simulink model "AB_Final_of_MPC_Bandwidth_Result_UnbalancedNew"  (R2022b)
settings: Solver=FixedStepDiscrete  StartTime=0.0  StopTime=Inf  FixedStep=100e-6  RelTol=1e-3  EnableMultiTasking=on
undefined symbols (not defined in the file): C28x, CPU1, CPU2, CurrentBypassValue, DiscIntNeverNeededParam, Down, GPTRIP1SEL, TZ1, Up
libraries: c2802xlib x20, simulink x17, dspstat3 x13, eeGeneralControl x10, c2837xDlib x5, c280xlib x5, PID_Lib x4, c2000lib x1, spsAlphaBetaZerotoabcLib x1
(part 7 of 10)

== system AB_Final_of_MPC_Bandwidth_Result_UnbalancedNew/Subsystem1/dq_abc1/Subsystem6 ==
  In1 : Inport
  In2 : Inport  Port=2
  theta : Inport  Port=3
  Add{,1,3..4} (4 alike) : Sum  Inputs=+-
  Add2 : Sum
  Constant : Constant  Value=2*pi/3
  Cos : Trigonometry  Operator=cos
  Cos1 : Trigonometry
  Cos2 : Trigonometry  Operator=cos
  Cos3 : Trigonometry
  Cos4 : Trigonometry
  Cos5 : Trigonometry  Operator=cos
  Product{,1..5} (6 alike) : Product
  Ia : Outport
  Ib : Outport  Port=2
  Ic : Outport  Port=3
  wires:
  theta/1 -> Add2/2, Add3/1, Cos1/1, Cos/1
  In1/1 -> [d]
  In2/1 -> [q]
  [d] -> Product/1
  Cos/1 -> [cosine]
  Cos1/1 -> [sinee]
  [cosine] -> Product/2
  [q] -> Product1/1
  [sinee] -> Product1/2
  Product/1 -> Add/1
  Product1/1 -> Add/2
  Add/1 -> Ia/1
  Constant/1 -> Add3/2, Add2/1
  Add2/1 -> Cos4/1, Cos2/1
  Add3/1 -> Cos5/1, Cos3/1
  Add1/1 -> Ib/1
  [d] -> Product2/1
  Cos3/1 -> Product3/2
  Product3/1 -> Add1/2
  [q] -> Product3/1
  Product2/1 -> Add1/1
  Cos5/1 -> Product2/2
  [q] -> Product5/1
  [d] -> Product4/1
  Product4/1 -> Add4/1
  Add4/1 -> Ic/1
  Cos4/1 -> Product5/2
  Product5/1 -> Add4/2
  Cos2/1 -> Product4/2

== system AB_Final_of_MPC_Bandwidth_Result_UnbalancedNew/Subsystem3/PLL_Loop2/ABCtoAlphaBeta ==
  In1 : Inport
  In2 : Inport  Port=2
  In3 : Inport  Port=3
  Add : Sum  Inputs=+-
  Add1 : Sum  Inputs=+--
  Gain : Gain  Gain=0.5
  Gain1 : Gain  Gain=sqrt(3)/2
  Gain2 : Gain  Gain=2/3
  Gain3 : Gain  Gain=2/3
  Gain4 : Gain  Gain=0.5
  Out1 : Outport
  Vαβ : Outport  Port=2
  wires:
  In1/1 -> Add1/1
  Gain4/1 -> Add1/3
  Gain/1 -> Add1/2
  In2/1 -> Add/1, Gain/1
  In3/1 -> Add/2, Gain4/1
  Add/1 -> Gain1/1
  Add1/1 -> Gain2/1
  Gain2/1 -> Out1/1
  Gain1/1 -> Gain3/1
  Gain3/1 -> Vαβ/1

== system AB_Final_of_MPC_Bandwidth_Result_UnbalancedNew/Subsystem3/PLL_Loop2/Discrete integrator 2π wrapping1 ==
  ω : Inport
  Compare To Constant : simulink/Logic and Bit Operations/Compare To Constant  relop=<  const=0  OutDataTypeStr=boolean
  Compare To Constant1 : simulink/Logic and Bit Operations/Compare To Constant  relop=>=  const=2*pi  OutDataTypeStr=boolean
  Discrete-Time Integrator : DiscreteIntegrator  ExternalReset=sampled level  InitialConditionSource=external  SampleTime=-1  ShowStatePort=on  ICPrevOutput=DiscIntNeverNeededParam  ICPrevScaledInput=DiscIntNeverNeededParam
  Gain : Gain  Gain=1/(2*pi)
      settings: AttributesFormatString=%<Gain>
  Gain1 : Gain  Gain=2*pi
  IC : InitialCondition  Value=0
  Logical Operator : Logic  Operator=OR  AllPortsSameDT=off  OutDataTypeStr=boolean
  Rounding Function : Rounding
  Sum1 : Sum  Inputs=|+-
  θ : Outport
  wires:
  Gain1/1 -> Sum1/2
  Gain/1 -> Rounding Function/1
  IC/1 -> Discrete-Time Integrator/3
  Compare To Constant1/1 -> Logical Operator/2
  Discrete-Time Integrator/State -> Compare To Constant1/1, Sum1/1, Gain/1, Compare To Constant/1
  Compare To Constant/1 -> Logical Operator/1
  Logical Operator/1 -> Discrete-Time Integrator/2
  Sum1/1 -> IC/1
  Rounding Function/1 -> Gain1/1
  ω/1 -> Discrete-Time Integrator/1
  Discrete-Time Integrator/1 -> θ/1

== system AB_Final_of_MPC_Bandwidth_Result_UnbalancedNew/Subsystem3/PLL_Loop2/SOGI 1st2 ==
  w : Inport
  Vαβ : Inport  Port=2
  Cast To Single : DataTypeConversion  OutDataTypeStr=single  SaturateOnIntegerOverflow=off  RndMeth=Floor
  Delay One Step : Delay  DelayLength=1  InitialCondition=0.5
  Delay One Step1 : Delay  DelayLength=1  InitialCondition=-0.5
  Gain : Gain  Gain=sqrt(2)  OutDataTypeStr=single
  Gain1 : Gain  Gain=100e-6  OutDataTypeStr=single
  Multiply1 : Product
  Product : Product
  Sum : Sum  Inputs=-+|
  Sum1 : Sum  Inputs=|+-
  Sum2 : Sum  Inputs=++|
  Sum3 : Sum  Inputs=++|
  v : Outport
  qv : Outport  Port=2  OutDataTypeStr=single
  wires:
  Sum/1 -> Gain/1
  Gain/1 -> Sum1/1
  Vαβ/1 -> Sum/2
  w/1 -> Gain1/1
  Sum1/1 -> Product/2
  Gain1/1 -> [WTs], Product/1
  Product/1 -> Sum2/2
  Sum2/1 -> Cast To Single/1, Delay One Step/1, v/1
  Delay One Step/1 -> Sum2/1, Sum/1
  [WTs] -> Multiply1/2
  Multiply1/1 -> Sum3/2
  Delay One Step1/1 -> Sum3/1, Sum1/2
  Sum3/1 -> Delay One Step1/1, qv/1
  Cast To Single/1 -> Multiply1/1

== system AB_Final_of_MPC_Bandwidth_Result_UnbalancedNew/Subsystem3/PLL_Loop2/SOGI 1st3 ==
  w : Inport
  Vαβ : Inport  Port=2
  Gain : Gain  Gain=sqrt(2)  OutDataTypeStr=single
  Gain1 : Gain  Gain=0  OutDataTypeStr=single
  Integrator : Subsystem
  Integrator1 : Subsystem
  Integrator2 : Subsystem
  Multiply : Product
  Multiply1 : Product
  Multiply2 : Product
  Saturation : Saturate  UpperLimit=5  LowerLimit=-5
  Sum : Sum  Inputs=-+|
  Sum1 : Sum  Inputs=|+-
  Sum2 : Sum  Inputs=++|
  v : Outport
  qv : Outport  Port=2  OutDataTypeStr=single
  wires:
  w/1 -> Multiply2/2, Multiply/2, Multiply1/1
  Sum/1 -> Saturation/1, Gain/1
  Gain/1 -> Sum1/1
  Vαβ/1 -> Sum/2
  Sum1/1 -> Multiply/1
  Multiply/1 -> Integrator/1(In)
  Multiply2/1 -> Integrator2/1(In)
  Gain1/1 -> Multiply2/1
  Saturation/1 -> Gain1/1
  Integrator/1(Out) -> Sum2/2, v/1, Integrator1/1(In)
  Integrator1/1(Out) -> Multiply1/2
  Multiply1/1 -> Sum1/2, qv/1
  Integrator2/1(Out) -> Sum2/1
  Sum2/1 -> Sum/1

== system AB_Final_of_MPC_Bandwidth_Result_UnbalancedNew/Subsystem3/PLL_Loop2/SOGI 1st4 ==
  w : Inport
  Vαβ : Inport  Port=2
  Cast To Single : DataTypeConversion  OutDataTypeStr=single  SaturateOnIntegerOverflow=off  RndMeth=Floor
  Delay One Step : Delay  DelayLength=1  InitialCondition=0.5
  Delay One Step1 : Delay  DelayLength=1  InitialCondition=-0.5
  Gain : Gain  Gain=sqrt(2)  OutDataTypeStr=single
  Gain1 : Gain  Gain=100e-6  OutDataTypeStr=single
  Multiply1 : Product
  Product : Product
  Sum : Sum  Inputs=-+|
  Sum1 : Sum  Inputs=|+-
  Sum2 : Sum  Inputs=++|
  Sum3 : Sum  Inputs=++|
  v : Outport
  qv : Outport  Port=2  OutDataTypeStr=single
  wires:
  Sum/1 -> Gain/1
  Gain/1 -> Sum1/1
  Vαβ/1 -> Sum/2
  w/1 -> Gain1/1
  Sum1/1 -> Product/2
  Gain1/1 -> [WTs], Product/1
  Product/1 -> Sum2/2
  Sum2/1 -> Cast To Single/1, Delay One Step/1, v/1
  Delay One Step/1 -> Sum2/1, Sum/1
  [WTs] -> Multiply1/2
  Multiply1/1 -> Sum3/2
  Delay One Step1/1 -> Sum3/1, Sum1/2
  Sum3/1 -> Delay One Step1/1, qv/1
  Cast To Single/1 -> Multiply1/1

== system AB_Final_of_MPC_Bandwidth_Result_UnbalancedNew/Subsystem3/PLL_Loop2/SOGI 1st5 ==
  w : Inport
  Vαβ : Inport  Port=2
  Gain : Gain  Gain=sqrt(2)  OutDataTypeStr=single
  Gain1 : Gain  Gain=0  OutDataTypeStr=single
  Integrator : Subsystem
  Integrator1 : Subsystem
  Integrator2 : Subsystem
  Multiply : Product
  Multiply1 : Product
  Multiply2 : Product
  Saturation : Saturate  UpperLimit=5  LowerLimit=-5
  Sum : Sum  Inputs=-+|
  Sum1 : Sum  Inputs=|+-
  Sum2 : Sum  Inputs=++|
  v : Outport
  qv : Outport  Port=2  OutDataTypeStr=single
  wires:
  w/1 -> Multiply2/2, Multiply/2, Multiply1/1
  Sum/1 -> Saturation/1, Gain/1
  Gain/1 -> Sum1/1
  Vαβ/1 -> Sum/2
  Sum1/1 -> Multiply/1
  Multiply/1 -> Integrator/1(In)
  Multiply2/1 -> Integrator2/1(In)
  Gain1/1 -> Multiply2/1
  Saturation/1 -> Gain1/1
  Integrator/1(Out) -> Sum2/2, v/1, Integrator1/1(In)
  Integrator1/1(Out) -> Multiply1/2
  Multiply1/1 -> Sum1/2, qv/1
  Integrator2/1(Out) -> Sum2/1
  Sum2/1 -> Sum/1

== system AB_Final_of_MPC_Bandwidth_Result_UnbalancedNew/Subsystem3/PLL_Loop2/Subsystem6 ==
  In1 : Inport
  In2 : Inport  Port=2
  theta : Inport  Port=3
  Add : Sum
  Add1 : Sum  Inputs=-+
  Cos : Trigonometry  Operator=cos
  Cos1 : Trigonometry
  From : From
  From4 : From
  Goto : Goto
  Product{,1..3} (4 alike) : Product
  Id : Outport
  Iq : Outport  Port=2
  wires:
  theta/1 -> Cos1/1, Cos/1
  In1/1 -> Goto/1
  In2/1 -> [b]
  From/1 -> Product/1
  Cos/1 -> [cosine]
  Cos1/1 -> [sinee]
  [cosine] -> Product/2
  [b] -> Product1/1
  [sinee] -> Product1/2
  Product/1 -> Add/1
  Product1/1 -> Add/2
  Add/1 -> Id/1
  [sinee] -> Product2/2
  [b] -> Product3/1
  Product3/1 -> Add1/2
  From4/1 -> Product2/1
  Product2/1 -> Add1/1
  [cosine] -> Product3/2
  Add1/1 -> Iq/1

== system AB_Final_of_MPC_Bandwidth_Result_UnbalancedNew/Voltage_Loop/Subsystem5/LPF ==
  u_k : Inport
  Add : Sum  Inputs=+-
  Add1 : Sum
  Delay : Delay  DelayLength=1
  Gain : Gain  Gain=single(1000/11000)
  y_k : Outport
  wires:
  Delay/1 -> Add/2, Add1/2
  Add/1 -> Gain/1
  Gain/1 -> Add1/1
  Add1/1 -> y_k/1, Delay/1
  u_k/1 -> Add/1

== system AB_Final_of_MPC_Bandwidth_Result_UnbalancedNew/Subsystem1/ABCtoDQO/abc_dq/Subsystem5 ==
  In1 : Inport
  In2 : Inport  Port=2
  In3 : Inport  Port=3
  Add : Sum  Inputs=+-
  Add1 : Sum  Inputs=+--
  Gain : Gain  Gain=0.5
  Gain1 : Gain  Gain=sqrt(3)/2
  Gain2 : Gain  Gain=2/3
  Gain3 : Gain  Gain=2/3
  Gain4 : Gain  Gain=0.5
  Id : Outport
  Iq : Outport  Port=2
  wires:
  In1/1 -> Add1/1
  Gain4/1 -> Add1/3
  Gain/1 -> Add1/2
  In2/1 -> Add/1, Gain/1
  In3/1 -> Add/2, Gain4/1
  Add/1 -> Gain1/1
  Add1/1 -> Gain2/1
  Gain2/1 -> Id/1
  Gain1/1 -> Gain3/1
  Gain3/1 -> Iq/1

== system AB_Final_of_MPC_Bandwidth_Result_UnbalancedNew/Subsystem1/ABCtoDQO/abc_dq1/Subsystem5 ==
  In1 : Inport
  In2 : Inport  Port=2
  In3 : Inport  Port=3
  Add : Sum  Inputs=+-
  Add1 : Sum  Inputs=+--
  Gain : Gain  Gain=0.5
  Gain1 : Gain  Gain=sqrt(3)/2
  Gain2 : Gain  Gain=2/3
  Gain3 : Gain  Gain=2/3
  Gain4 : Gain  Gain=0.5
  Id : Outport
  Iq : Outport  Port=2
  wires:
  In1/1 -> Add1/1
  Gain4/1 -> Add1/3
  Gain/1 -> Add1/2
  In2/1 -> Add/1, Gain/1
  In3/1 -> Add/2, Gain4/1
  Add/1 -> Gain1/1
  Add1/1 -> Gain2/1
  Gain2/1 -> Id/1
  Gain1/1 -> Gain3/1
  Gain3/1 -> Iq/1

== system AB_Final_of_MPC_Bandwidth_Result_UnbalancedNew/Subsystem1/AlphaBetaDutiesCalculation/DutiesCalculation/Duty_Sector1 ==
  MPCC_f32AlphaVoltageReference : Inport
  MPCC_f32BetaVoltageReference : Inport  Port=2
  MPCC_f32AlphaConvVoltage1 : Inport  Port=3
  MPCC_f32AlphaConvVoltage2 : Inport  Port=4
  MPCC_f32BetaConvVoltage1 : Inport  Port=5
  MPCC_f32BetaConvVoltage2 : Inport  Port=6
  Add : Sum  Inputs=+--
  Constant : Constant  Value=single(1)
  DutyA_Sector1 : Subsystem
  DutyB_Sector1 : Subsystem
  Mux : Mux  Inputs=3
  Mux1 : Mux  Inputs=2
  SectorNumber : Constant  Value=single(1)
  Signal Copy : SignalConversion  OverrideOpt=off
  MPCC_f32Duty_Sector1 : Outport
  wires:
  MPCC_f32AlphaVoltageReference/1 -> [MPCC_f32AlphaVoltageReference]
  MPCC_f32BetaVoltageReference/1 -> [MPCC_f32BetaVoltageReference]
  MPCC_f32AlphaConvVoltage1/1 -> [MPCC_f32AlphaConvVoltage1]
  MPCC_f32BetaConvVoltage1/1 -> [MPCC_f32BetaConvVoltage1]
  MPCC_f32AlphaConvVoltage2/1 -> [MPCC_f32AlphaConvVoltage2]
  MPCC_f32BetaConvVoltage2/1 -> [MPCC_f32BetaConvVoltage2]
  SectorNumber/1 -> Signal Copy/1
  Signal Copy/1 -> [MPCC_u8SectorNumber]
  DutyA_Sector1/1(MPCC_f32DutyA_Sector1) -> [MPCC_f32DutyA_Sector1]
  [MPCC_f32AlphaVoltageReference] -> DutyA_Sector1/1(MPCC_f32AlphaVoltageReference)
  [MPCC_f32BetaVoltageReference] -> DutyA_Sector1/2(MPCC_f32BetaVoltageReference)
  [MPCC_f32AlphaConvVoltage1] -> DutyA_Sector1/3(MPCC_f32AlphaConvVoltage1)
  [MPCC_f32AlphaConvVoltage2] -> DutyA_Sector1/4(MPCC_f32AlphaConvVoltage2)
  [MPCC_f32BetaConvVoltage1] -> DutyA_Sector1/5(MPCC_f32BetaConvVoltage1)
  [MPCC_f32BetaConvVoltage2] -> DutyA_Sector1/6(MPCC_f32BetaConvVoltage2)
  [MPCC_f32BetaVoltageReference] -> DutyB_Sector1/2(MPCC_f32BetaVoltageReference)
  [MPCC_f32AlphaConvVoltage1] -> DutyB_Sector1/3(MPCC_f32AlphaConvVoltage1)
  [MPCC_f32AlphaVoltageReference] -> DutyB_Sector1/1(MPCC_f32AlphaVoltageReference)
  [MPCC_f32AlphaConvVoltage2] -> DutyB_Sector1/4(MPCC_f32AlphaConvVoltage2)
  [MPCC_f32BetaConvVoltage1] -> DutyB_Sector1/5(MPCC_f32BetaConvVoltage1)
  DutyB_Sector1/1(MPCC_f32DutyB_Sector1) -> [MPCC_f32DutyB_Sector1]
  [MPCC_f32BetaConvVoltage2] -> DutyB_Sector1/6(MPCC_f32BetaConvVoltage2)
  Constant/1 -> Add/1
  Add/1 -> [MPCC_f32DutyO_Sector1]
  [MPCC_f32DutyB_Sector1] -> Add/3
  [MPCC_f32DutyA_Sector1] -> Add/2
  [MPCC_f32DutyA_Sector1] -> Mux/1
  [MPCC_f32DutyB_Sector1] -> Mux/2
  [MPCC_f32DutyO_Sector1] -> Mux/3
  Mux/1 -> Mux1/1
  [MPCC_u8SectorNumber] -> Mux1/2
  Mux1/1 -> MPCC_f32Duty_Sector1/1

== system AB_Final_of_MPC_Bandwidth_Result_UnbalancedNew/Subsystem1/AlphaBetaDutiesCalculation/DutiesCalculation/Duty_Sector2 ==
  MPCC_f32AlphaVoltageReference : Inport
  MPCC_f32BetaVoltageReference : Inport  Port=2
  MPCC_f32AlphaConvVoltage2 : Inport  Port=3
  MPCC_f32AlphaConvVoltage3 : Inport  Port=4
  MPCC_f32BetaConvVoltage2 : Inport  Port=5
  MPCC_f32BetaConvVoltage3 : Inport  Port=6
  Add : Sum  Inputs=+--
  Constant : Constant  Value=single(1)
  DutyA_Sector2 : Subsystem
  DutyB_Sector2 : Subsystem
  Mux : Mux  Inputs=3
  Mux1 : Mux  Inputs=2
  SectorNumber : Constant  Value=single(2)
  Signal Copy : SignalConversion  OverrideOpt=off
  MPCC_f32Duty_Sector2 : Outport
  wires:
  MPCC_f32AlphaVoltageReference/1 -> [MPCC_f32AlphaVoltageReference]
  MPCC_f32BetaVoltageReference/1 -> [MPCC_f32BetaVoltageReference]
  MPCC_f32AlphaConvVoltage2/1 -> [MPCC_f32AlphaConvVoltage2]
  MPCC_f32BetaConvVoltage2/1 -> [MPCC_f32BetaConvVoltage2]
  MPCC_f32AlphaConvVoltage3/1 -> [MPCC_f32AlphaConvVoltage3]
  MPCC_f32BetaConvVoltage3/1 -> [MPCC_f32BetaConvVoltage3]
  SectorNumber/1 -> Signal Copy/1
  Signal Copy/1 -> [MPCC_u8SectorNumber]
  DutyA_Sector2/1(MPCC_f32DutyA_Sector2) -> [MPCC_f32DutyA_Sector2]
  [MPCC_f32AlphaVoltageReference] -> DutyA_Sector2/1(MPCC_f32AlphaVoltageReference)
  [MPCC_f32BetaVoltageReference] -> DutyA_Sector2/2(MPCC_f32BetaVoltageReference)
  [MPCC_f32AlphaConvVoltage2] -> DutyA_Sector2/3(MPCC_f32AlphaConvVoltage2)
  [MPCC_f32AlphaConvVoltage3] -> DutyA_Sector2/4(MPCC_f32AlphaConvVoltage3)
  [MPCC_f32BetaConvVoltage2] -> DutyA_Sector2/5(MPCC_f32BetaConvVoltage2)
  [MPCC_f32BetaConvVoltage3] -> DutyA_Sector2/6(MPCC_f32BetaConvVoltage3)
  [MPCC_f32BetaVoltageReference] -> DutyB_Sector2/2(MPCC_f32BetaVoltageReference)
  [MPCC_f32AlphaVoltageReference] -> DutyB_Sector2/1(MPCC_f32AlphaVoltageReference)
  DutyB_Sector2/1(MPCC_f32DutyB_Sector2) -> [MPCC_f32DutyB_Sector2]
  Constant/1 -> Add/1
  Add/1 -> [MPCC_f32DutyO_Sector2]
  [MPCC_f32DutyB_Sector2] -> Add/3
  [MPCC_f32DutyA_Sector2] -> Add/2
  [MPCC_f32DutyA_Sector2] -> Mux/1
  [MPCC_f32DutyB_Sector2] -> Mux/2
  [MPCC_f32DutyO_Sector2] -> Mux/3
  Mux/1 -> Mux1/1
  [MPCC_u8SectorNumber] -> Mux1/2
  Mux1/1 -> MPCC_f32Duty_Sector2/1
  [MPCC_f32AlphaConvVoltage2] -> DutyB_Sector2/3(MPCC_f32AlphaConvVoltage2)
  [MPCC_f32BetaConvVoltage3] -> DutyB_Sector2/6(MPCC_f32BetaConvVoltage3)
  [MPCC_f32AlphaConvVoltage3] -> DutyB_Sector2/4(MPCC_f32AlphaConvVoltage3)
  [MPCC_f32BetaConvVoltage2] -> DutyB_Sector2/5(MPCC_f32BetaConvVoltage2)

== system AB_Final_of_MPC_Bandwidth_Result_UnbalancedNew/Subsystem1/AlphaBetaDutiesCalculation/DutiesCalculation/Duty_Sector3 ==
  MPCC_f32AlphaVoltageReference : Inport
  MPCC_f32BetaVoltageReference : Inport  Port=2
  MPCC_f32AlphaConvVoltage3 : Inport  Port=3
  MPCC_f32AlphaConvVoltage4 : Inport  Port=4
  MPCC_f32BetaConvVoltage3 : Inport  Port=5
  MPCC_f32BetaConvVoltage4 : Inport  Port=6
  Add : Sum  Inputs=+--
  Constant : Constant  Value=single(1)
  DutyA_Sector3 : Subsystem
  DutyB_Sector3 : Subsystem
  Mux : Mux  Inputs=3
  Mux1 : Mux  Inputs=2
  SectorNumber : Constant  Value=single(3)
  Signal Copy : SignalConversion  OverrideOpt=off
  MPCC_f32Duty_Sector3 : Outport
  wires:
  MPCC_f32AlphaVoltageReference/1 -> [MPCC_f32AlphaVoltageReference]
  MPCC_f32BetaVoltageReference/1 -> [MPCC_f32BetaVoltageReference]
  SectorNumber/1 -> Signal Copy/1
  Signal Copy/1 -> [MPCC_u8SectorNumber]
  DutyA_Sector3/1(MPCC_f32DutyA_Sector3) -> [MPCC_f32DutyA_Sector3]
  [MPCC_f32AlphaVoltageReference] -> DutyA_Sector3/1(MPCC_f32AlphaVoltageReference)
  [MPCC_f32BetaVoltageReference] -> DutyA_Sector3/2(MPCC_f32BetaVoltageReference)
  [MPCC_f32AlphaConvVoltage3] -> DutyA_Sector3/3(MPCC_f32AlphaConvVoltage3)
  [MPCC_f32AlphaConvVoltage4] -> DutyA_Sector3/4(MPCC_f32AlphaConvVoltage4)
  [MPCC_f32BetaConvVoltage3] -> DutyA_Sector3/5(MPCC_f32BetaConvVoltage3)
  [MPCC_f32BetaConvVoltage4] -> DutyA_Sector3/6(MPCC_f32BetaConvVoltage4)
  DutyB_Sector3/1(MPCC_f32DutyB_Sector3) -> [MPCC_f32DutyB_Sector3]
  Constant/1 -> Add/1
  Add/1 -> [MPCC_f32DutyO_Sector3]
  [MPCC_f32DutyB_Sector3] -> Add/3
  [MPCC_f32DutyA_Sector3] -> Add/2
  [MPCC_f32DutyA_Sector3] -> Mux/1
  [MPCC_f32DutyB_Sector3] -> Mux/2
  [MPCC_f32DutyO_Sector3] -> Mux/3
  Mux/1 -> Mux1/1
  [MPCC_u8SectorNumber] -> Mux1/2
  Mux1/1 -> MPCC_f32Duty_Sector3/1
  [MPCC_f32AlphaVoltageReference] -> DutyB_Sector3/1(MPCC_f32AlphaVoltageReference)
  [MPCC_f32AlphaConvVoltage3] -> DutyB_Sector3/3(MPCC_f32AlphaConvVoltage3)
  [MPCC_f32BetaConvVoltage4] -> DutyB_Sector3/6(MPCC_f32BetaConvVoltage4)
  [MPCC_f32BetaVoltageReference] -> DutyB_Sector3/2(MPCC_f32BetaVoltageReference)
  [MPCC_f32AlphaConvVoltage4] -> DutyB_Sector3/4(MPCC_f32AlphaConvVoltage4)
  [MPCC_f32BetaConvVoltage3] -> DutyB_Sector3/5(MPCC_f32BetaConvVoltage3)
  MPCC_f32AlphaConvVoltage3/1 -> [MPCC_f32AlphaConvVoltage3]
  MPCC_f32BetaConvVoltage4/1 -> [MPCC_f32BetaConvVoltage4]
  MPCC_f32AlphaConvVoltage4/1 -> [MPCC_f32AlphaConvVoltage4]
  MPCC_f32BetaConvVoltage3/1 -> [MPCC_f32BetaConvVoltage3]

== system AB_Final_of_MPC_Bandwidth_Result_UnbalancedNew/Subsystem1/AlphaBetaDutiesCalculation/DutiesCalculation/Duty_Sector4 ==
  MPCC_f32AlphaVoltageReference : Inport
  MPCC_f32BetaVoltageReference : Inport  Port=2
  MPCC_f32AlphaConvVoltage4 : Inport  Port=3
  MPCC_f32AlphaConvVoltage5 : Inport  Port=4
  MPCC_f32BetaConvVoltage4 : Inport  Port=5
  MPCC_f32BetaConvVoltage5 : Inport  Port=6
  Add : Sum  Inputs=+--
  Constant : Constant  Value=single(1)
  DutyA_Sector4 : Subsystem
  DutyB_Sector4 : Subsystem
  Mux : Mux  Inputs=3
  Mux1 : Mux  Inputs=2
  SectorNumber : Constant  Value=single(4)
  Signal Copy : SignalConversion  OverrideOpt=off
  MPCC_f32Duty_Sector4 : Outport
  wires:
  MPCC_f32AlphaVoltageReference/1 -> [MPCC_f32AlphaVoltageReference]
  MPCC_f32BetaVoltageReference/1 -> [MPCC_f32BetaVoltageReference]
  SectorNumber/1 -> Signal Copy/1
  Signal Copy/1 -> [MPCC_u8SectorNumber]
  DutyA_Sector4/1(MPCC_f32DutyA_Sector4) -> [MPCC_f32DutyA_Sector4]
  [MPCC_f32AlphaVoltageReference] -> DutyA_Sector4/1(MPCC_f32AlphaVoltageReference)
  [MPCC_f32BetaVoltageReference] -> DutyA_Sector4/2(MPCC_f32BetaVoltageReference)
  [MPCC_f32AlphaConvVoltage4] -> DutyA_Sector4/3(MPCC_f32AlphaConvVoltage4)
  [MPCC_f32AlphaConvVoltage5] -> DutyA_Sector4/4(MPCC_f32AlphaConvVoltage5)
  [MPCC_f32BetaConvVoltage4] -> DutyA_Sector4/5(MPCC_f32BetaConvVoltage4)
  [MPCC_f32BetaConvVoltage5] -> DutyA_Sector4/6(MPCC_f32BetaConvVoltage5)
  DutyB_Sector4/1(MPCC_f32DutyB_Sector4) -> [MPCC_f32DutyB_Sector4]
  Constant/1 -> Add/1
  Add/1 -> [MPCC_f32DutyO_Sector4]
  [MPCC_f32DutyB_Sector4] -> Add/3
  [MPCC_f32DutyA_Sector4] -> Add/2
  [MPCC_f32DutyA_Sector4] -> Mux/1
  [MPCC_f32DutyB_Sector4] -> Mux/2
  [MPCC_f32DutyO_Sector4] -> Mux/3
  Mux/1 -> Mux1/1
  [MPCC_u8SectorNumber] -> Mux1/2
  Mux1/1 -> MPCC_f32Duty_Sector4/1
  MPCC_f32BetaConvVoltage5/1 -> [MPCC_f32BetaConvVoltage5]
  MPCC_f32BetaConvVoltage4/1 -> [MPCC_f32BetaConvVoltage4]
  MPCC_f32AlphaConvVoltage4/1 -> [MPCC_f32AlphaConvVoltage4]
  MPCC_f32AlphaConvVoltage5/1 -> [MPCC_f32AlphaConvVoltage5]
  [MPCC_f32AlphaVoltageReference] -> DutyB_Sector4/1(MPCC_f32AlphaVoltageReference)
  [MPCC_f32AlphaConvVoltage4] -> DutyB_Sector4/3(MPCC_f32AlphaConvVoltage4)
  [MPCC_f32BetaConvVoltage5] -> DutyB_Sector4/6(MPCC_f32BetaConvVoltage5)
  [MPCC_f32BetaVoltageReference] -> DutyB_Sector4/2(MPCC_f32BetaVoltageReference)
  [MPCC_f32AlphaConvVoltage5] -> DutyB_Sector4/4(MPCC_f32AlphaConvVoltage5)
  [MPCC_f32BetaConvVoltage4] -> DutyB_Sector4/5(MPCC_f32BetaConvVoltage4)

== system AB_Final_of_MPC_Bandwidth_Result_UnbalancedNew/Subsystem1/AlphaBetaDutiesCalculation/DutiesCalculation/Duty_Sector5 ==
  MPCC_f32AlphaVoltageReference : Inport
  MPCC_f32BetaVoltageReference : Inport  Port=2
  MPCC_f32AlphaConvVoltage5 : Inport  Port=3
  MPCC_f32AlphaConvVoltage6 : Inport  Port=4
  MPCC_f32BetaConvVoltage5 : Inport  Port=5
  MPCC_f32BetaConvVoltage6 : Inport  Port=6
  Add : Sum  Inputs=+--
  Constant : Constant  Value=single(1)
  DutyA_Sector5 : Subsystem
  DutyB_Sector5 : Subsystem
  Mux : Mux  Inputs=3
  Mux1 : Mux  Inputs=2
  SectorNumber : Constant  Value=single(5)
  Signal Copy : SignalConversion  OverrideOpt=off
  MPCC_f32Duty_Sector5 : Outport
  wires:
  MPCC_f32AlphaVoltageReference/1 -> [MPCC_f32AlphaVoltageReference]
  MPCC_f32BetaVoltageReference/1 -> [MPCC_f32BetaVoltageReference]
  SectorNumber/1 -> Signal Copy/1
  Signal Copy/1 -> [MPCC_u8SectorNumber]
  DutyA_Sector5/1(MPCC_f32DutyA_Sector5) -> [MPCC_f32DutyA_Sector5]
  [MPCC_f32AlphaVoltageReference] -> DutyA_Sector5/1(MPCC_f32AlphaVoltageReference)
  [MPCC_f32BetaVoltageReference] -> DutyA_Sector5/2(MPCC_f32BetaVoltageReference)
  [MPCC_f32AlphaConvVoltage5] -> DutyA_Sector5/3(MPCC_f32AlphaConvVoltage5)
  [MPCC_f32AlphaConvVoltage6] -> DutyA_Sector5/4(MPCC_f32AlphaConvVoltage6)
  [MPCC_f32BetaConvVoltage5] -> DutyA_Sector5/5(MPCC_f32BetaConvVoltage5)
  [MPCC_f32BetaConvVoltage6] -> DutyA_Sector5/6(MPCC_f32BetaConvVoltage6)
  DutyB_Sector5/1(MPCC_f32DutyB_Sector5) -> [MPCC_f32DutyB_Sector5]
  Constant/1 -> Add/1
  Add/1 -> [MPCC_f32DutyO_Sector5]
  [MPCC_f32DutyB_Sector5] -> Add/3
  [MPCC_f32DutyA_Sector5] -> Add/2
  [MPCC_f32DutyA_Sector5] -> Mux/1
  [MPCC_f32DutyB_Sector5] -> Mux/2
  [MPCC_f32DutyO_Sector5] -> Mux/3
  Mux/1 -> Mux1/1
  [MPCC_u8SectorNumber] -> Mux1/2
  Mux1/1 -> MPCC_f32Duty_Sector5/1
  MPCC_f32BetaConvVoltage6/1 -> [MPCC_f32BetaConvVoltage6]
  MPCC_f32AlphaConvVoltage5/1 -> [MPCC_f32AlphaConvVoltage5]
  MPCC_f32BetaConvVoltage5/1 -> [MPCC_f32BetaConvVoltage5]
  MPCC_f32AlphaConvVoltage6/1 -> [MPCC_f32AlphaConvVoltage6]
  [MPCC_f32AlphaVoltageReference] -> DutyB_Sector5/1(MPCC_f32AlphaVoltageReference)
  [MPCC_f32AlphaConvVoltage5] -> DutyB_Sector5/3(MPCC_f32AlphaConvVoltage5)
  [MPCC_f32BetaConvVoltage6] -> DutyB_Sector5/6(MPCC_f32BetaConvVoltage6)
  [MPCC_f32BetaVoltageReference] -> DutyB_Sector5/2(MPCC_f32BetaVoltageReference)
  [MPCC_f32AlphaConvVoltage6] -> DutyB_Sector5/4(MPCC_f32AlphaConvVoltage6)
  [MPCC_f32BetaConvVoltage5] -> DutyB_Sector5/5(MPCC_f32BetaConvVoltage5)

== system AB_Final_of_MPC_Bandwidth_Result_UnbalancedNew/Subsystem1/AlphaBetaDutiesCalculation/DutiesCalculation/Duty_Sector6 ==
  MPCC_f32AlphaVoltageReference : Inport
  MPCC_f32BetaVoltageReference : Inport  Port=2
  MPCC_f32AlphaConvVoltage6 : Inport  Port=3
  MPCC_f32AlphaConvVoltage1 : Inport  Port=4
  MPCC_f32BetaConvVoltage6 : Inport  Port=5
  MPCC_f32BetaConvVoltage1 : Inport  Port=6
  Add : Sum  Inputs=+--
  Constant : Constant  Value=single(1)
  DutyA_Sector6 : Subsystem
  DutyB_Sector6 : Subsystem
  Mux : Mux  Inputs=3
  Mux1 : Mux  Inputs=2
  SectorNumber : Constant  Value=single(6)
  Signal Copy : SignalConversion  OverrideOpt=off
  MPCC_f32Duty_Sector6 : Outport
  wires:
  MPCC_f32AlphaVoltageReference/1 -> [MPCC_f32AlphaVoltageReference]
  MPCC_f32BetaVoltageReference/1 -> [MPCC_f32BetaVoltageReference]
  SectorNumber/1 -> Signal Copy/1
  Signal Copy/1 -> [MPCC_u8SectorNumber]
  DutyA_Sector6/1(MPCC_f32DutyA_Sector6) -> [MPCC_f32DutyA_Sector6]
  [MPCC_f32AlphaVoltageReference] -> DutyA_Sector6/1(MPCC_f32AlphaVoltageReference)
  [MPCC_f32BetaVoltageReference] -> DutyA_Sector6/2(MPCC_f32BetaVoltageReference)
  [MPCC_f32AlphaConvVoltage6] -> DutyA_Sector6/3(MPCC_f32AlphaConvVoltage6)
  [MPCC_f32AlphaConvVoltage1] -> DutyA_Sector6/4(MPCC_f32AlphaConvVoltage1)
  [MPCC_f32BetaConvVoltage6] -> DutyA_Sector6/5(MPCC_f32BetaConvVoltage6)
  [MPCC_f32BetaConvVoltage1] -> DutyA_Sector6/6(MPCC_f32BetaConvVoltage1)
  DutyB_Sector6/1(MPCC_f32DutyB_Sector6) -> [MPCC_f32DutyB_Sector6]
  Constant/1 -> Add/1
  Add/1 -> [MPCC_f32DutyO_Sector6]
  [MPCC_f32DutyB_Sector6] -> Add/3
  [MPCC_f32DutyA_Sector6] -> Add/2
  [MPCC_f32DutyA_Sector6] -> Mux/1
  [MPCC_f32DutyB_Sector6] -> Mux/2
  [MPCC_f32DutyO_Sector6] -> Mux/3
  Mux/1 -> Mux1/1
  [MPCC_u8SectorNumber] -> Mux1/2
  Mux1/1 -> MPCC_f32Duty_Sector6/1
  MPCC_f32BetaConvVoltage1/1 -> [MPCC_f32BetaConvVoltage1]
  MPCC_f32AlphaConvVoltage6/1 -> [MPCC_f32AlphaConvVoltage6]
  MPCC_f32BetaConvVoltage6/1 -> [MPCC_f32BetaConvVoltage6]
  MPCC_f32AlphaConvVoltage1/1 -> [MPCC_f32AlphaConvVoltage1]
  [MPCC_f32AlphaVoltageReference] -> DutyB_Sector6/1(MPCC_f32AlphaVoltageReference)
  [MPCC_f32AlphaConvVoltage6] -> DutyB_Sector6/3(MPCC_f32AlphaConvVoltage6)
  [MPCC_f32BetaConvVoltage1] -> DutyB_Sector6/6(MPCC_f32BetaConvVoltage1)
  [MPCC_f32BetaVoltageReference] -> DutyB_Sector6/2(MPCC_f32BetaVoltageReference)
  [MPCC_f32AlphaConvVoltage1] -> DutyB_Sector6/4(MPCC_f32AlphaConvVoltage1)
  [MPCC_f32BetaConvVoltage6] -> DutyB_Sector6/5(MPCC_f32BetaConvVoltage6)

== system AB_Final_of_MPC_Bandwidth_Result_UnbalancedNew/Subsystem1/Decoupling_Loop/ABCtoDQOVoltage/DQOtoA ==
  PI_f32MDVoltageRef : Inport
  PI_f32MQVoltageRef : Inport  Port=2
  PI_f32MOVoltageRef : Inport  Port=3
  PI_f32ElectricalAngle : Inport  Port=4
  Add : Sum  Inputs=+++  OutDataTypeStr=single
  Constant1 : Constant  Value=single(1)
  Gain : Gain  Gain=single(1)
  Gain1 : Gain  Gain=single(1)
  Product : Product
  Product1 : Product
  Product2 : Product
  Saturation1 : Saturate  UpperLimit=1  LowerLimit=-1  ZeroCross=off
  Sin1 : Trigonometry  Operator=cos
  Sin3 : Trigonometry
  PI_f32MAVoltageRef : Outport
  wires:
  Sin1/1 -> Product1/2
  PI_f32ElectricalAngle/1 -> [PI_f32ElectricalAngle]
  Product1/1 -> Gain1/1
  Product2/1 -> Add/3
  Product/1 -> Add/1
  Constant1/1 -> Product2/2
  [PI_f32ElectricalAngle] -> Sin1/1
  Add/1 -> Gain/1
  PI_f32MQVoltageRef/1 -> Product1/1
  [PI_f32ElectricalAngle] -> Sin3/1
  PI_f32MDVoltageRef/1 -> Product/1
  Sin3/1 -> Product/2
  PI_f32MOVoltageRef/1 -> Product2/1
  Gain/1 -> Saturation1/1
  Saturation1/1 -> PI_f32MAVoltageRef/1
  Gain1/1 -> Add/2

== system AB_Final_of_MPC_Bandwidth_Result_UnbalancedNew/Subsystem1/Decoupling_Loop/ABCtoDQOVoltage/DQOtoB ==
  PI_f32MDVoltageRef : Inport
  PI_f32MQVoltageRef : Inport  Port=2
  PI_f32MOVoltageRef : Inport  Port=3
  PI_f32ElectricalAngle : Inport  Port=4
  Add : Sum  Inputs=+++  OutDataTypeStr=single
  Add1 : Sum  Inputs=+-
  Add3 : Sum  Inputs=+-
  Constant : Constant  Value=single(2*pi/3)
  Constant1 : Constant  Value=single(1)
  Constant2 : Constant  Value=single(2*pi/3)
  Gain : Gain  Gain=single(1)
  Gain1 : Gain  Gain=single(1)
  Product : Product
  Product1 : Product
  Product2 : Product
  Saturation1 : Saturate  UpperLimit=1  LowerLimit=-1  ZeroCross=off
  Sin1 : Trigonometry  Operator=cos
  Sin3 : Trigonometry
  PI_f32MBVoltageRef : Outport
  wires:
  Sin1/1 -> Product1/2
  PI_f32ElectricalAngle/1 -> [PI_f32ElectricalAngle]
  Product1/1 -> Gain1/1
  Constant/1 -> Add1/2
  Product2/1 -> Add/3
  Product/1 -> Add/1
  Constant1/1 -> Product2/2
  Add1/1 -> Sin1/1
  Add/1 -> Gain/1
  [PI_f32ElectricalAngle] -> Add1/1
  PI_f32MQVoltageRef/1 -> Product1/1
  PI_f32MDVoltageRef/1 -> Product/1
  Sin3/1 -> Product/2
  PI_f32MOVoltageRef/1 -> Product2/1
  Gain/1 -> Saturation1/1
  Constant2/1 -> Add3/2
  [PI_f32ElectricalAngle] -> Add3/1
  Add3/1 -> Sin3/1
  Saturation1/1 -> PI_f32MBVoltageRef/1
  Gain1/1 -> Add/2

== system AB_Final_of_MPC_Bandwidth_Result_UnbalancedNew/Subsystem1/Decoupling_Loop/ABCtoDQOVoltage/DQOtoC ==
  PI_f32MDVoltageRef : Inport
  PI_f32MQVoltageRef : Inport  Port=2
  PI_f32MOVoltageRef : Inport  Port=3
  PI_f32ElectricalAngle : Inport  Port=4
  Add : Sum  Inputs=+++  OutDataTypeStr=single
  Add1 : Sum
  Add3 : Sum
  Constant : Constant  Value=single(2*pi/3)
  Constant1 : Constant  Value=single(1)
  Constant2 : Constant  Value=single(2*pi/3)
  Gain : Gain  Gain=single(1)
  Gain1 : Gain  Gain=single(1)
  Product : Product  OutDataTypeStr=Inherit: Inherit via back propagation
  Product1 : Product  OutDataTypeStr=Inherit: Inherit via back propagation
  Product2 : Product  OutDataTypeStr=Inherit: Inherit via back propagation
  Saturation1 : Saturate  UpperLimit=1  LowerLimit=-1  ZeroCross=off
  Sin1 : Trigonometry  Operator=cos
  Sin3 : Trigonometry
  PI_f32MCVoltageRef : Outport
  wires:
  Sin1/1 -> Product1/2
  PI_f32ElectricalAngle/1 -> [PI_f32ElectricalAngle]
  Product1/1 -> Gain1/1
  Constant/1 -> Add1/2
  Product2/1 -> Add/3
  Product/1 -> Add/1
  Constant1/1 -> Product2/2
  Add1/1 -> Sin1/1
  Add/1 -> Gain/1
  [PI_f32ElectricalAngle] -> Add1/1
  PI_f32MQVoltageRef/1 -> Product1/1
  PI_f32MDVoltageRef/1 -> Product/1
  Sin3/1 -> Product/2
  PI_f32MOVoltageRef/1 -> Product2/1
  Gain/1 -> Saturation1/1
  Constant2/1 -> Add3/2
  [PI_f32ElectricalAngle] -> Add3/1
  Add3/1 -> Sin3/1
  Saturation1/1 -> PI_f32MCVoltageRef/1
  Gain1/1 -> Add/2

== system AB_Final_of_MPC_Bandwidth_Result_UnbalancedNew/Subsystem1/Decoupling_Loop/dq_abc/Subsystem6 ==
  In1 : Inport
  In2 : Inport  Port=2
  theta : Inport  Port=3
  Add{,1,3..4} (4 alike) : Sum  Inputs=+-
  Add2 : Sum
  Constant : Constant  Value=2*pi/3
  Cos : Trigonometry  Operator=cos
  Cos1 : Trigonometry
  Cos2 : Trigonometry  Operator=cos
  Cos3 : Trigonometry
  Cos4 : Trigonometry
  Cos5 : Trigonometry  Operator=cos
  Product{,1..5} (6 alike) : Product
  Ia : Outport
  Ib : Outport  Port=2
  Ic : Outport  Port=3
  wires:
  theta/1 -> Add2/2, Add3/1, Cos1/1, Cos/1
  In1/1 -> [d]
  In2/1 -> [q]
  [d] -> Product/1
  Cos/1 -> [cosine]
  Cos1/1 -> [sinee]
  [cosine] -> Product/2
  [q] -> Product1/1
  [sinee] -> Product1/2
  Product/1 -> Add/1
  Product1/1 -> Add/2
  Add/1 -> Ia/1
  Constant/1 -> Add3/2, Add2/1
  Add2/1 -> Cos4/1, Cos2/1
  Add3/1 -> Cos5/1, Cos3/1
  Add1/1 -> Ib/1
  [d] -> Product2/1
  Cos3/1 -> Product3/2
  Product3/1 -> Add1/2
  [q] -> Product3/1
  Product2/1 -> Add1/1
  Cos5/1 -> Product2/2
  [q] -> Product5/1
  [d] -> Product4/1
  Product4/1 -> Add4/1
  Add4/1 -> Ic/1
  Cos4/1 -> Product5/2
  Product5/1 -> Add4/2
  Cos2/1 -> Product4/2

== system AB_Final_of_MPC_Bandwidth_Result_UnbalancedNew/Subsystem1/GridCurrentSecondPrediction/CostFunctionofSectors/Duty_Sector1 ==
  MPCC_f32CostFunction_Voltage1 : Inport
  MPCC_f32CostFunction_Voltage2 : Inport  Port=2
  MPCC_f32Duty_Sector1 : Inport  Port=3
  Abs : Abs  SaturateOnIntegerOverflow=off
  Abs1 : Abs  SaturateOnIntegerOverflow=off
  Add3 : Sum
  Demux : Demux
  Product4 : Product
  Product5 : Product
  MPCC_f32CostFunction_Sector1 : Outport
  wires:
  Demux/2 -> [MPCC_f32DutyB_Sector1]
  MPCC_f32Duty_Sector1/1 -> Demux/1
  Demux/1 -> [MPCC_f32DutyA_Sector1]
  MPCC_f32CostFunction_Voltage1/1 -> Product4/1
  [MPCC_f32DutyA_Sector1] -> Product4/2
  MPCC_f32CostFunction_Voltage2/1 -> Product5/1
  [MPCC_f32DutyB_Sector1] -> Product5/2
  Product4/1 -> Abs/1
  Product5/1 -> Abs1/1
  Add3/1 -> MPCC_f32CostFunction_Sector1/1
  Abs/1 -> Add3/1
  Abs1/1 -> Add3/2

== system AB_Final_of_MPC_Bandwidth_Result_UnbalancedNew/Subsystem1/GridCurrentSecondPrediction/CostFunctionofSectors/Duty_Sector2 ==
  MPCC_f32CostFunction_Voltage2 : Inport
  MPCC_f32CostFunction_Voltage3 : Inport  Port=2
  MPCC_f32Duty_Sector2 : Inport  Port=3
  Abs1 : Abs  SaturateOnIntegerOverflow=off
  Abs2 : Abs  SaturateOnIntegerOverflow=off
  Add3 : Sum
  Demux : Demux
  Product4 : Product
  Product5 : Product
  MPCC_f32CostFunction_Sector2 : Outport
  wires:
  MPCC_f32CostFunction_Voltage2/1 -> Product4/1
  [MPCC_f32DutyA_Sector2] -> Product4/2
  MPCC_f32CostFunction_Voltage3/1 -> Product5/1
  [MPCC_f32DutyB_Sector2] -> Product5/2
  Product4/1 -> Abs1/1
  Product5/1 -> Abs2/1
  Add3/1 -> MPCC_f32CostFunction_Sector2/1
  Abs1/1 -> Add3/1
  Abs2/1 -> Add3/2
  Demux/1 -> [MPCC_f32DutyA_Sector2]
  Demux/2 -> [MPCC_f32DutyB_Sector2]
  MPCC_f32Duty_Sector2/1 -> Demux/1

== system AB_Final_of_MPC_Bandwidth_Result_UnbalancedNew/Subsystem1/GridCurrentSecondPrediction/CostFunctionofSectors/Duty_Sector3 ==
  MPCC_f32CostFunction_Voltage3 : Inport
  MPCC_f32CostFunction_Voltage4 : Inport  Port=2
  MPCC_f32Duty_Sector3 : Inport  Port=3
  Abs : Abs  SaturateOnIntegerOverflow=off
  Abs1 : Abs  SaturateOnIntegerOverflow=off
  Add3 : Sum
  Demux : Demux
  Product4 : Product
  Product5 : Product
  MPCC_f32CostFunction_Sector3 : Outport
  wires:
  Demux/2 -> [MPCC_f32DutyB_Sector3]
  Demux/1 -> [MPCC_f32DutyA_Sector3]
  MPCC_f32CostFunction_Voltage3/1 -> Product4/1
  [MPCC_f32DutyA_Sector3] -> Product4/2
  MPCC_f32CostFunction_Voltage4/1 -> Product5/1
  [MPCC_f32DutyB_Sector3] -> Product5/2
  Product4/1 -> Abs/1
  Product5/1 -> Abs1/1
  Add3/1 -> MPCC_f32CostFunction_Sector3/1
  Abs/1 -> Add3/1
  Abs1/1 -> Add3/2
  MPCC_f32Duty_Sector3/1 -> Demux/1

== system AB_Final_of_MPC_Bandwidth_Result_UnbalancedNew/Subsystem1/GridCurrentSecondPrediction/CostFunctionofSectors/Duty_Sector4 ==
  MPCC_f32CostFunction_Voltage4 : Inport
  MPCC_f32CostFunction_Voltage5 : Inport  Port=2
  MPCC_f32Duty_Sector4 : Inport  Port=3
  Abs1 : Abs  SaturateOnIntegerOverflow=off
  Abs2 : Abs  SaturateOnIntegerOverflow=off
  Add3 : Sum
  Demux : Demux
  Product4 : Product
  Product5 : Product
  MPCC_f32CostFunction_Sector4 : Outport
  wires:
  MPCC_f32CostFunction_Voltage4/1 -> Product4/1
  [MPCC_f32DutyA_Sector4] -> Product4/2
  MPCC_f32CostFunction_Voltage5/1 -> Product5/1
  [MPCC_f32DutyB_Sector4] -> Product5/2
  Product4/1 -> Abs1/1
  Product5/1 -> Abs2/1
  Add3/1 -> MPCC_f32CostFunction_Sector4/1
  Abs1/1 -> Add3/1
  Abs2/1 -> Add3/2
  MPCC_f32Duty_Sector4/1 -> Demux/1
  Demux/1 -> [MPCC_f32DutyA_Sector4]
  Demux/2 -> [MPCC_f32DutyB_Sector4]

== system AB_Final_of_MPC_Bandwidth_Result_UnbalancedNew/Subsystem1/GridCurrentSecondPrediction/CostFunctionofSectors/Duty_Sector5 ==
  MPCC_f32CostFunction_Voltage5 : Inport
  MPCC_f32CostFunction_Voltage6 : Inport  Port=2
  MPCC_f32Duty_Sector5 : Inport  Port=3
  Abs1 : Abs  SaturateOnIntegerOverflow=off
  Abs2 : Abs  SaturateOnIntegerOverflow=off
  Add3 : Sum
  Demux : Demux
  Product4 : Product
  Product5 : Product
  MPCC_f32CostFunction_Sector5 : Outport
  wires:
  MPCC_f32CostFunction_Voltage5/1 -> Product4/1
  [MPCC_f32DutyA_Sector5] -> Product4/2
  MPCC_f32CostFunction_Voltage6/1 -> Product5/1
  [MPCC_f32DutyB_Sector5] -> Product5/2
  Product4/1 -> Abs1/1
  Product5/1 -> Abs2/1
  Add3/1 -> MPCC_f32CostFunction_Sector5/1
  Abs1/1 -> Add3/1
  Abs2/1 -> Add3/2
  MPCC_f32Duty_Sector5/1 -> Demux/1
  Demux/1 -> [MPCC_f32DutyA_Sector5]
  Demux/2 -> [MPCC_f32DutyB_Sector5]

== system AB_Final_of_MPC_Bandwidth_Result_UnbalancedNew/Subsystem1/GridCurrentSecondPrediction/CostFunctionofSectors/Duty_Sector6 ==
  MPCC_f32CostFunction_Voltage6 : Inport
  MPCC_f32CostFunction_Voltage1 : Inport  Port=2
  MPCC_f32Duty_Sector6 : Inport  Port=3
  Abs1 : Abs  SaturateOnIntegerOverflow=off
  Abs2 : Abs  SaturateOnIntegerOverflow=off
  Add3 : Sum
  Demux : Demux
  Product4 : Product
  Product5 : Product
  MPCC_f32CostFunction_Sector6 : Outport
  wires:
  MPCC_f32CostFunction_Voltage6/1 -> Product4/1
  [MPCC_f32DutyA_Sector6] -> Product4/2
  MPCC_f32CostFunction_Voltage1/1 -> Product5/1
  [MPCC_f32DutyB_Sector6] -> Product5/2
  Product4/1 -> Abs1/1
  Product5/1 -> Abs2/1
  Add3/1 -> MPCC_f32CostFunction_Sector6/1
  Abs1/1 -> Add3/1
  Abs2/1 -> Add3/2
  MPCC_f32Duty_Sector6/1 -> Demux/1
  Demux/1 -> [MPCC_f32DutyA_Sector6]
  Demux/2 -> [MPCC_f32DutyB_Sector6]

== system AB_Final_of_MPC_Bandwidth_Result_UnbalancedNew/Subsystem1/GridCurrentSecondPrediction/CostFunctionofVoltageVectors/CostFunctionVoltage1 ==
  MPCC_f32DGridCurrent_K_1 : Inport
  MPCC_f32QGridCurrent_K_1 : Inport  Port=2
  MPCC_f32DGridVoltage : Inport  Port=3
  MPCC_f32QGridVoltage : Inport  Port=4
  MPCC_f32Predictionterm_A : Inport  Port=5
  MPCC_f32Predictionterm_B : Inport  Port=6
  MPCC_f32Predictionterm_C : Inport  Port=7
  MPCC_f32DGridCurrentReference : Inport  Port=8
  MPCC_f32QGridCurrentReference : Inport  Port=9
  MPCC_f32DVoltageVector1 : Inport  Port=10
  MPCC_f32QVoltageVector1 : Inport  Port=11
  MPCC_f32DGridCurrent : Inport  Port=12
  MPCC_f32QGridCurrent : Inport  Port=13
  MPCC_f32DGridCurrent1 : Inport  Port=14
  MPCC_f32QGridCurrent1 : Inport  Port=15
  CostFunctionVoltage1 : Subsystem
  DGridCurrentSecondPrediction_Voltage1 : Subsystem
  QGridCurrentSecondPrediction_Voltage1 : Subsystem
  MPCC_f32CostFunction_Voltage1 : Outport
  wires:
  [MPCC_f32Predictionterm_B] -> QGridCurrentSecondPrediction_Voltage1/2(MPCC_f32Predictionterm_B)
  [MPCC_f32QGridCurrent_K_1] -> DGridCurrentSecondPrediction_Voltage1/5(MPCC_f32QGridCurrent_K_1)
  [MPCC_f32Predictionterm_A] -> QGridCurrentSecondPrediction_Voltage1/1(MPCC_f32Predictionterm_A)
  [MPCC_f32QGridCurrent_K_1] -> QGridCurrentSecondPrediction_Voltage1/5(MPCC_f32QGridCurrent_K_1)
  [MPCC_f32Predictionterm_B] -> DGridCurrentSecondPrediction_Voltage1/2(MPCC_f32Predictionterm_B)
  [MPCC_f32DGridCurrent_K_1] -> QGridCurrentSecondPrediction_Voltage1/4(MPCC_f32DGridCurrent_K_1)
  [MPCC_f32Predictionterm_C] -> QGridCurrentSecondPrediction_Voltage1/3(MPCC_f32Predictionterm_C)
  [MPCC_f32Predictionterm_A] -> DGridCurrentSecondPrediction_Voltage1/1(MPCC_f32Predictionterm_A)
  DGridCurrentSecondPrediction_Voltage1/1(MPCC_f32DGridCurrent_K_2_Voltage1) -> [MPCC_f32DGridCurrent_K_2_Voltage1]
  [MPCC_f32Predictionterm_C] -> DGridCurrentSecondPrediction_Voltage1/3(MPCC_f32Predictionterm_C)
  [MPCC_f32QGridVoltage] -> QGridCurrentSecondPrediction_Voltage1/6(MPCC_f32QGridVoltage)
  [MPCC_f32DGridVoltage] -> DGridCurrentSecondPrediction_Voltage1/6(MPCC_f32DGridVoltage)
  [MPCC_f32DGridCurrent_K_1] -> DGridCurrentSecondPrediction_Voltage1/4(MPCC_f32DGridCurrent_K_1)
  MPCC_f32QGridVoltage/1 -> [MPCC_f32QGridVoltage]
  MPCC_f32DGridCurrent_K_1/1 -> [MPCC_f32DGridCurrent_K_1]
  MPCC_f32Predictionterm_A/1 -> [MPCC_f32Predictionterm_A]
  MPCC_f32DGridVoltage/1 -> [MPCC_f32DGridVoltage]
  MPCC_f32Predictionterm_C/1 -> [MPCC_f32Predictionterm_C]
  MPCC_f32QGridCurrent_K_1/1 -> [MPCC_f32QGridCurrent_K_1]
  MPCC_f32Predictionterm_B/1 -> [MPCC_f32Predictionterm_B]
  MPCC_f32DGridCurrentReference/1 -> [MPCC_f32DGridCurrentReference]
  MPCC_f32QGridCurrentReference/1 -> [MPCC_f32QGridCurrentReference]
  QGridCurrentSecondPrediction_Voltage1/1(MPCC_f32QGridCurrent_K_2_Voltage1) -> [MPCC_f32QGridCurrent_K_2_Voltage1]
  CostFunctionVoltage1/1(MPCC_f32CostFunction_Voltage1) -> MPCC_f32CostFunction_Voltage1/1
  [MPCC_f32DGridCurrentReference] -> CostFunctionVoltage1/1(MPCC_f32DGridCurrentReference)
  [MPCC_f32QGridCurrentReference] -> CostFunctionVoltage1/2(MPCC_f32QGridCurrentReference)
  [MPCC_f32DGridCurrent_K_2_Voltage1] -> CostFunctionVoltage1/3(MPCC_f32DGridCurrent_K_2_Voltage1)
  [MPCC_f32QGridCurrent_K_2_Voltage1] -> CostFunctionVoltage1/4(MPCC_f32QGridCurrent_K_2_Voltage1)
  [MPCC_f32DGridCurrent] -> CostFunctionVoltage1/5(MPCC_f32DGridCurrent)
  [MPCC_f32QGridCurrent] -> CostFunctionVoltage1/6(MPCC_f32QGridCurrent)
  [MPCC_f32DVoltageVector1] -> DGridCurrentSecondPrediction_Voltage1/7(MPCC_f32DVoltageVector1)
  [MPCC_f32QVoltageVector1] -> QGridCurrentSecondPrediction_Voltage1/7(MPCC_f32QVoltageVector1)
  MPCC_f32DVoltageVector1/1 -> [MPCC_f32DVoltageVector1]
  MPCC_f32QVoltageVector1/1 -> [MPCC_f32QVoltageVector1]
  MPCC_f32DGridCurrent/1 -> [MPCC_f32DGridCurrent]
  MPCC_f32QGridCurrent/1 -> [MPCC_f32QGridCurrent]
  MPCC_f32DGridCurrent1/1 -> CostFunctionVoltage1/7(MPCC_f32DGridCurrent1)
  MPCC_f32QGridCurrent1/1 -> CostFunctionVoltage1/8(MPCC_f32QGridCurrent1)

== system AB_Final_of_MPC_Bandwidth_Result_UnbalancedNew/Subsystem1/GridCurrentSecondPrediction/CostFunctionofVoltageVectors/CostFunctionVoltage2 ==
  MPCC_f32DGridCurrent_K_1 : Inport
  MPCC_f32QGridCurrent_K_1 : Inport  Port=2
  MPCC_f32DGridVoltage : Inport  Port=3
  MPCC_f32QGridVoltage : Inport  Port=4
  MPCC_f32Predictionterm_A : Inport  Port=5
  MPCC_f32Predictionterm_B : Inport  Port=6
  MPCC_f32Predictionterm_C : Inport  Port=7
  MPCC_f32DGridCurrentReference : Inport  Port=8
  MPCC_f32QGridCurrentReference : Inport  Port=9
  MPCC_f32DVoltageVector2 : Inport  Port=10
  MPCC_f32QVoltageVector2 : Inport  Port=11
  MPCC_f32DGridCurrent : Inport  Port=12
  MPCC_f32QGridCurrent : Inport  Port=13
  MPCC_f32DGridCurrent1 : Inport  Port=14
  MPCC_f32QGridCurrent1 : Inport  Port=15
  CostFunctionVoltage2 : Subsystem
  DGridCurrentSecondPrediction_Voltage2 : Subsystem
  QGridCurrentSecondPrediction_Voltage2 : Subsystem
  MPCC_f32CostFunction_Voltage2 : Outport
  wires:
  [MPCC_f32Predictionterm_B] -> QGridCurrentSecondPrediction_Voltage2/2(MPCC_f32Predictionterm_B)
  [MPCC_f32QGridCurrent_K_1] -> DGridCurrentSecondPrediction_Voltage2/5(MPCC_f32QGridCurrent_K_1)
  [MPCC_f32Predictionterm_A] -> QGridCurrentSecondPrediction_Voltage2/1(MPCC_f32Predictionterm_A)
  [MPCC_f32QGridCurrent_K_1] -> QGridCurrentSecondPrediction_Voltage2/5(MPCC_f32QGridCurrent_K_1)
  [MPCC_f32Predictionterm_B] -> DGridCurrentSecondPrediction_Voltage2/2(MPCC_f32Predictionterm_B)
  [MPCC_f32DGridCurrent_K_1] -> QGridCurrentSecondPrediction_Voltage2/4(MPCC_f32DGridCurrent_K_1)
  [MPCC_f32Predictionterm_C] -> QGridCurrentSecondPrediction_Voltage2/3(MPCC_f32Predictionterm_C)
  [MPCC_f32Predictionterm_A] -> DGridCurrentSecondPrediction_Voltage2/1(MPCC_f32Predictionterm_A)
  DGridCurrentSecondPrediction_Voltage2/1(MPCC_f32DGridCurrent_K_2_Voltage2) -> [MPCC_f32DGridCurrent_K_2_Voltage2]
  [MPCC_f32Predictionterm_C] -> DGridCurrentSecondPrediction_Voltage2/3(MPCC_f32Predictionterm_C)
  [MPCC_f32QGridVoltage] -> QGridCurrentSecondPrediction_Voltage2/6(MPCC_f32QGridVoltage)
  [MPCC_f32DGridVoltage] -> DGridCurrentSecondPrediction_Voltage2/6(MPCC_f32DGridVoltage)
  [MPCC_f32DGridCurrent_K_1] -> DGridCurrentSecondPrediction_Voltage2/4(MPCC_f32DGridCurrent_K_1)
  MPCC_f32QGridVoltage/1 -> [MPCC_f32QGridVoltage]
  MPCC_f32DGridCurrent_K_1/1 -> [MPCC_f32DGridCurrent_K_1]
  MPCC_f32Predictionterm_A/1 -> [MPCC_f32Predictionterm_A]
  MPCC_f32DGridVoltage/1 -> [MPCC_f32DGridVoltage]
  MPCC_f32Predictionterm_C/1 -> [MPCC_f32Predictionterm_C]
  MPCC_f32QGridCurrent_K_1/1 -> [MPCC_f32QGridCurrent_K_1]
  MPCC_f32Predictionterm_B/1 -> [MPCC_f32Predictionterm_B]
  MPCC_f32DGridCurrentReference/1 -> [MPCC_f32DGridCurrentReference]
  MPCC_f32QGridCurrentReference/1 -> [MPCC_f32QGridCurrentReference]
  QGridCurrentSecondPrediction_Voltage2/1(MPCC_f32QGridCurrent_K_2_Voltage2) -> [MPCC_f32QGridCurrent_K_2_Voltage2]
  CostFunctionVoltage2/1(MPCC_f32CostFunction_Voltage2) -> MPCC_f32CostFunction_Voltage2/1
  [MPCC_f32DGridCurrentReference] -> CostFunctionVoltage2/1(MPCC_f32DGridCurrentReference)
  [MPCC_f32QGridCurrentReference] -> CostFunctionVoltage2/2(MPCC_f32QGridCurrentReference)
  [MPCC_f32DGridCurrent_K_2_Voltage2] -> CostFunctionVoltage2/3(MPCC_f32DGridCurrent_K_2_Voltage2)
  [MPCC_f32QGridCurrent_K_2_Voltage2] -> CostFunctionVoltage2/4(MPCC_f32QGridCurrent_K_2_Voltage2)
  [MPCC_f32DGridCurrent] -> CostFunctionVoltage2/5(MPCC_f32DGridCurrent)
  [MPCC_f32QGridCurrent] -> CostFunctionVoltage2/6(MPCC_f32QGridCurrent)
  [MPCC_f32DVoltageVector2] -> DGridCurrentSecondPrediction_Voltage2/7(MPCC_f32DVoltageVector2)
  [MPCC_f32QVoltageVector2] -> QGridCurrentSecondPrediction_Voltage2/7(MPCC_f32QVoltageVector2)
  MPCC_f32DVoltageVector2/1 -> [MPCC_f32DVoltageVector2]
  MPCC_f32QVoltageVector2/1 -> [MPCC_f32QVoltageVector2]
  MPCC_f32QGridCurrent/1 -> [MPCC_f32QGridCurrent]
  MPCC_f32DGridCurrent/1 -> [MPCC_f32DGridCurrent]
  MPCC_f32DGridCurrent1/1 -> CostFunctionVoltage2/7(MPCC_f32DGridCurrent1)
  MPCC_f32QGridCurrent1/1 -> CostFunctionVoltage2/8(MPCC_f32QGridCurrent1)

== system AB_Final_of_MPC_Bandwidth_Result_UnbalancedNew/Subsystem1/GridCurrentSecondPrediction/CostFunctionofVoltageVectors/CostFunctionVoltage3 ==
  MPCC_f32DGridCurrent_K_1 : Inport
  MPCC_f32QGridCurrent_K_1 : Inport  Port=2
  MPCC_f32DGridVoltage : Inport  Port=3
  MPCC_f32QGridVoltage : Inport  Port=4
  MPCC_f32Predictionterm_A : Inport  Port=5
  MPCC_f32Predictionterm_B : Inport  Port=6
  MPCC_f32Predictionterm_C : Inport  Port=7
  MPCC_f32DGridCurrentReference : Inport  Port=8
  MPCC_f32QGridCurrentReference : Inport  Port=9
  MPCC_f32DVoltageVector3 : Inport  Port=10
  MPCC_f32QVoltageVector3 : Inport  Port=11
  MPCC_f32DGridCurrent : Inport  Port=12
  MPCC_f32QGridCurrent : Inport  Port=13
  MPCC_f32DGridCurrent1 : Inport  Port=14
  MPCC_f32QGridCurrent1 : Inport  Port=15
  CostFunctionVoltage3 : Subsystem
  DGridCurrentSecondPrediction_Voltage3 : Subsystem
  QGridCurrentSecondPrediction_Voltage3 : Subsystem
  MPCC_f32CostFunction_Voltage3 : Outport
  wires:
  [MPCC_f32Predictionterm_B] -> QGridCurrentSecondPrediction_Voltage3/2(MPCC_f32Predictionterm_B)
  [MPCC_f32QGridCurrent_K_1] -> DGridCurrentSecondPrediction_Voltage3/5(MPCC_f32QGridCurrent_K_1)
  [MPCC_f32Predictionterm_A] -> QGridCurrentSecondPrediction_Voltage3/1(MPCC_f32Predictionterm_A)
  [MPCC_f32QGridCurrent_K_1] -> QGridCurrentSecondPrediction_Voltage3/5(MPCC_f32QGridCurrent_K_1)
  [MPCC_f32Predictionterm_B] -> DGridCurrentSecondPrediction_Voltage3/2(MPCC_f32Predictionterm_B)
  [MPCC_f32DGridCurrent_K_1] -> QGridCurrentSecondPrediction_Voltage3/4(MPCC_f32DGridCurrent_K_1)
  [MPCC_f32Predictionterm_C] -> QGridCurrentSecondPrediction_Voltage3/3(MPCC_f32Predictionterm_C)
  [MPCC_f32Predictionterm_A] -> DGridCurrentSecondPrediction_Voltage3/1(MPCC_f32Predictionterm_A)
  DGridCurrentSecondPrediction_Voltage3/1(MPCC_f32DGridCurrent_K_2_Voltage3) -> [MPCC_f32DGridCurrent_K_2_Voltage3]
  [MPCC_f32Predictionterm_C] -> DGridCurrentSecondPrediction_Voltage3/3(MPCC_f32Predictionterm_C)
  [MPCC_f32QGridVoltage] -> QGridCurrentSecondPrediction_Voltage3/6(MPCC_f32QGridVoltage)
  [MPCC_f32DGridVoltage] -> DGridCurrentSecondPrediction_Voltage3/6(MPCC_f32DGridVoltage)
  [MPCC_f32DGridCurrent_K_1] -> DGridCurrentSecondPrediction_Voltage3/4(MPCC_f32DGridCurrent_K_1)
  MPCC_f32QGridVoltage/1 -> [MPCC_f32QGridVoltage]
  MPCC_f32DGridCurrent_K_1/1 -> [MPCC_f32DGridCurrent_K_1]
  MPCC_f32Predictionterm_A/1 -> [MPCC_f32Predictionterm_A]
  MPCC_f32DGridVoltage/1 -> [MPCC_f32DGridVoltage]
  MPCC_f32Predictionterm_C/1 -> [MPCC_f32Predictionterm_C]
  MPCC_f32QGridCurrent_K_1/1 -> [MPCC_f32QGridCurrent_K_1]
  MPCC_f32Predictionterm_B/1 -> [MPCC_f32Predictionterm_B]
  MPCC_f32DGridCurrentReference/1 -> [MPCC_f32DGridCurrentReference]
  MPCC_f32QGridCurrentReference/1 -> [MPCC_f32QGridCurrentReference]
  QGridCurrentSecondPrediction_Voltage3/1(MPCC_f32QGridCurrent_K_2_Voltage3) -> [MPCC_f32QGridCurrent_K_2_Voltage3]
  CostFunctionVoltage3/1(MPCC_f32CostFunction_Voltage3) -> MPCC_f32CostFunction_Voltage3/1
  [MPCC_f32DGridCurrentReference] -> CostFunctionVoltage3/1(MPCC_f32DGridCurrentReference)
  [MPCC_f32QGridCurrentReference] -> CostFunctionVoltage3/2(MPCC_f32QGridCurrentReference)
  [MPCC_f32DGridCurrent_K_2_Voltage3] -> CostFunctionVoltage3/3(MPCC_f32DGridCurrent_K_2_Voltage3)
  [MPCC_f32QGridCurrent_K_2_Voltage3] -> CostFunctionVoltage3/4(MPCC_f32QGridCurrent_K_2_Voltage3)
  [MPCC_f32DGridCurrent] -> CostFunctionVoltage3/5(MPCC_f32DGridCurrent)
  [MPCC_f32QGridCurrent] -> CostFunctionVoltage3/6(MPCC_f32QGridCurrent)
  [MPCC_f32DVoltageVector3] -> DGridCurrentSecondPrediction_Voltage3/7(MPCC_f32DVoltageVector3)
  [MPCC_f32QVoltageVector3] -> QGridCurrentSecondPrediction_Voltage3/7(MPCC_f32QVoltageVector3)
  MPCC_f32DVoltageVector3/1 -> [MPCC_f32DVoltageVector3]
  MPCC_f32QVoltageVector3/1 -> [MPCC_f32QVoltageVector3]
  MPCC_f32DGridCurrent/1 -> [MPCC_f32DGridCurrent]
  MPCC_f32QGridCurrent/1 -> [MPCC_f32QGridCurrent]
  MPCC_f32DGridCurrent1/1 -> CostFunctionVoltage3/7(MPCC_f32DGridCurrent1)
  MPCC_f32QGridCurrent1/1 -> CostFunctionVoltage3/8(MPCC_f32QGridCurrent1)
